simulink model "s0r0"  (R2019b)
settings: Solver=VariableStepAuto  StartTime=0.0  StopTime=10.0  RelTol=1e-3
values from neighbouring files (symbols this model uses):
  A = A*(v_phi(k,i)*s^i)    [Roberts_Q_design.m]    (also in main_fmincon.m = []; rocket_model.m = [0,1,0,0,0,0; ss_model.mat = [0  0; 1  0]; verif.m = [0,1;0,0])
  Aobs = A-L*C    [rocket_model.m]    (also in sim_controller_design.m)
  B = B*(s-alpha(i))    [Roberts_Q_design.m]    (also in controller_design.m = B*C(2); main_yp_fminunc.m = B*C(2); rocket_controllerdesign.m = B*C(2); rocket_controllerdesign_z.m = B*C(2))
  Bobs = [B L]    [rocket_model.m]    (also in sim_controller_design.m)
  C = [0,1]    [controller_design.m]    (also in main_yp_fminunc.m; rocket_controllerdesign.m; rocket_controllerdesign_z.m; rocket_model.m = eye(6))
  Cobs = eye(6)    [rocket_model.m]    (also in sim_controller_design.m = eye(2))
  Dobs = 0*Bobs    [rocket_model.m]    (also in sim_controller_design.m)
  K = minreal(Q/(1+Q*P))    [cost.m]    (also in cost_LQ.m = tf((conv(denQ{1},numK0{1})+conv(numQ{1},den_sys{1})),(conv(d; cost_con.m = tf((conv(denQ{1},numK0{1})+conv(numQ{1},den_sys{1})),(conv(d; cost_disturb.m = tf((conv(denQ{1},numK0{1})+conv(numQ{1},den_sys{1})),(conv(d; fminunc_LQ.m = tf((conv(denQ{1},numK0{1})+conv(numQ{1},den_sys{1})),(conv(d)
settings Model: Creator=bia  LastModifiedBy=bia
settings DataIOCC: LoadExternalInput=on

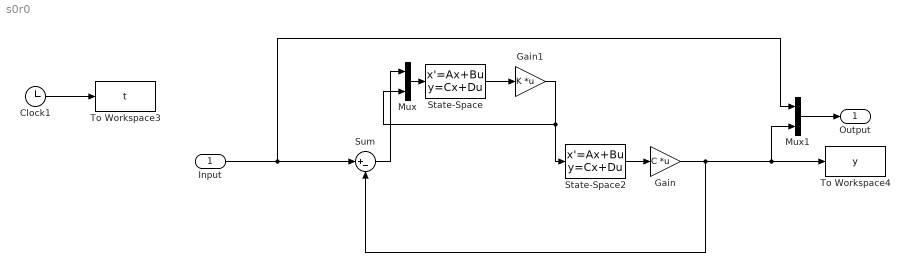
== system s0r0 ==
  Input : Inport
  Clock1 : Clock
  Gain : Gain  Gain=C  Multiplication=Matrix(K*u)
  Gain1 : Gain  Gain=K  Multiplication=Matrix(K*u)
  Mux : Mux  Inputs=2
  Mux1 : Mux  Inputs=2
  State-Space : StateSpace  A=Aobs  B=Bobs  C=Cobs  D=Dobs  InitialCondition=[0;0]
  State-Space2 : StateSpace  A=A  B=B  C=eye(2)  D=[0;0]  InitialCondition=[0;0]
  Sum : Sum  Inputs=|+-
  To Workspace3 : ToWorkspace  VariableName=t  SampleTime=-1
  To Workspace4 : ToWorkspace  VariableName=y  SampleTime=-1
  Output : Outport  SignalName=y
  wires:
  State-Space2/1 -> Gain/1
  Gain/1 -> Mux1/2, To Workspace4/1, Sum/2
  Clock1/1 -> To Workspace3/1
  Input/1 -> Mux1/1, Sum/1
  State-Space/1 -> Gain1/1
  Gain1/1 -> Mux/2, State-Space2/1
  Mux/1 -> State-Space/1
  Sum/1 -> Mux/1
  Mux1/1 -> Output/1
